simulink model "teng_sw_idc"  (R2016a)
settings: Solver=VariableStepAuto  StartTime=0.0  StopTime=5  RelTol=1e-3
libraries: fl_lib x7, elec_lib x5, nesl_utility x5, simulink x2
settings Model: Creator=mugino  LastModifiedBy=mugino
settings SolverCC: AlgebraicLoopSolver=LineSearch

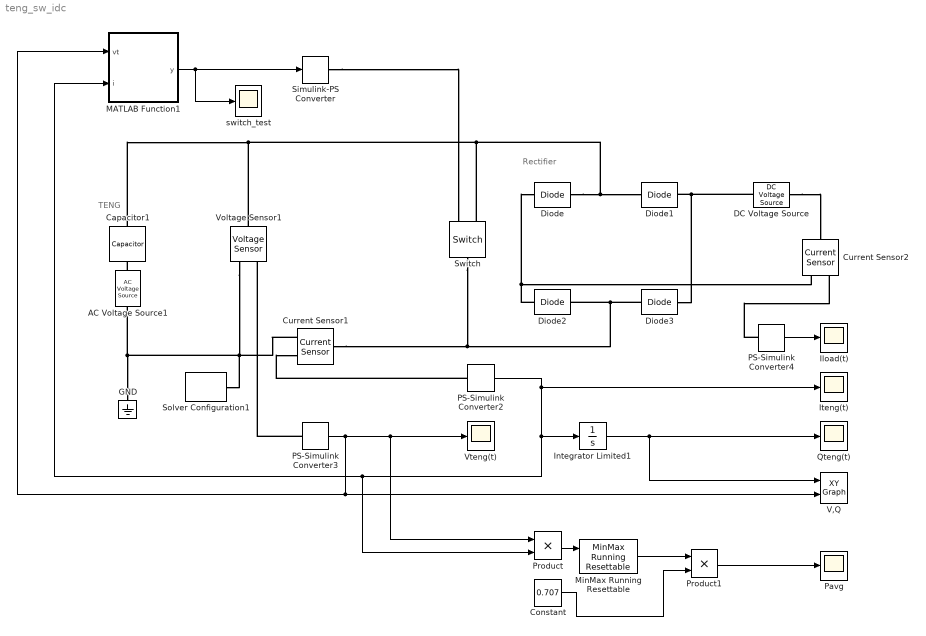
== system teng_sw_idc ==
  note: Rectifier
  note: TENG
  AC Voltage Source1 : fl_lib/Electrical/Electrical Sources/AC Voltage Source  amp=140 V  shift=90 deg  frequency=1 Hz  omega=0 rad/s
  Capacitor1 : elec_lib/Passive Devices/Capacitor  enable_table=0  c=2e-10 F  Cvec=[ 1e-5 1e-6 ] F  Vvec=[ 0 10 ] V  CV_table_symmetry=1  C_tol=5  enable_C_tol=0  tol_distribution=1  nSigma=4  r=60 MOhm  g=0 1/Ohm  initV=0 V  enable_operating_limits=0  operating_limit_action=2  max_working_voltage_range=[ -25 25 ] V  power_rating=1 W  enable_faults=0  fault_action=1  Cscale_faulted=100  R_faulted=0.001 Ohm  G_faulted=0 1/Ohm  tau_fault=0.001 s  enable_temporal_fault=0  t_fault=1 s  enable_behavioral_fault=0  max_permissible_voltage_range=[ -100 100 ] V  t_fail_on_voltage=1 s
  Constant : Constant  Value=0.707
  Current Sensor1 : fl_lib/Electrical/Electrical Sensors/Current Sensor
  Current Sensor2 : fl_lib/Electrical/Electrical Sensors/Current Sensor
  DC Voltage Source : fl_lib/Electrical/Electrical Sources/DC Voltage Source  v0=60 V
  Diode{,1..3} (4 alike) : elec_lib/Semiconductor Devices/Diode  ModelType=3  Vf=0.7 V  Ron=0.3 Ohm  Goff=1e-8 S  Rz=0.3 Ohm  Vz=50 V  C_PWL=5 pF  prmExp=1  I12=[ 0.0137 0.545 ] A  V12=[ 0.6 0.7 ] V  I1=0.0137 A  V1=0.6 V  RS=0.01 Ohm  IS=1e-12 A  Tmeas=25 degC  ec=1  BV=Inf V  C_param=1  CJ0=5 pF  VJ=1 V  Mgrad=0.5  Vvec=[ 0.1 10 100 ] V  Cvec=[ 3.5 1 0.4 ] pF  FC=0.5  Q_param=1  Irrm=-7.15 A  iF=4 A  didt=-750 A/us  trr=115 ns  TT=50 ns  tau=100 ns  T_param=1  IS_T2=1.25e-7 A  I1_T2=0.245 A  V1_T2=0.5 V  Tmeas2=125 degC  EG_param=1  EG=1.11 eV  XTI_param=1  XTI=3  dBVdT=0 V/K  Tdevice=25 degC  Rth=[ 0 10 ] K/W  thermal_mass_parameterization=1  thermal_mass=[ 0 1 ] J/K  thermal_time_constant=[ 0 10 ] s  thermal_mass_initial_temperatures=[ 25 25 ] degC
  GND : fl_lib/Electrical/Electrical Elements/Electrical Reference
  Iload(t) : Scope
  Integrator Limited1 : Integrator  LimitOutput=on  UpperSaturationLimit=1  LowerSaturationLimit=0
  Iteng(t) : Scope
  MATLAB Function1 : MATLAB Function  TreatAsAtomicUnit=on
  MinMax Running Resettable : simulink/Math Operations/MinMax Running Resettable  Function=max  vinit=0.0
  PS-Simulink Converter2 : nesl_utility/PS-Simulink Converter  PhysicalDomain=network_engine_domain  SubClassName=ps_output  LeftPortType=input  RightPortType=output  PseudoPeriodic=off  Frequencies=[]  Unit=A  AffineConversion=off
  PS-Simulink Converter3 : nesl_utility/PS-Simulink Converter  PhysicalDomain=network_engine_domain  SubClassName=ps_output  LeftPortType=input  RightPortType=output  PseudoPeriodic=off  Frequencies=[]  Unit=V  AffineConversion=off
  PS-Simulink Converter4 : nesl_utility/PS-Simulink Converter  PhysicalDomain=network_engine_domain  SubClassName=ps_output  LeftPortType=input  RightPortType=output  PseudoPeriodic=off  Frequencies=[]  Unit=A  AffineConversion=off
  "Pavg " : Scope
  Product : Product
  Product1 : Product
  Qteng(t) : Scope
  Simulink-PS Converter : nesl_utility/Simulink-PS Converter  PhysicalDomain=network_engine_domain  SubClassName=ps_input  LeftPortType=input  RightPortType=output  PseudoPeriodic=off  Frequencies=[]  NoiseDistribution=none  NoiseParameters=[]  Unit=1  AffineConversion=off  InputFiltering=off  SimscapeFilterOrder=1  InputFilterTimeConstant=0.001  UdotUserProvided=1
  Solver Configuration1 : nesl_utility/Solver Configuration  PhysicalDomain=network_engine_domain  SubClassName=solver  LeftPortType=input  RightPortType=generic  Accelerate=off  Tones=[]  Harmonics=[]  SimulateNoise=off  Profile=off  UseLocalSampling=off  EnableSwitchedLinearOptims=on  FrequencyDomain=off  UseCCode=off  RelTol=0.001  AbsTol=1e-06  MinStep=1e-09  ToWorkspace=off  RevertToSquareIcSolve=off  NumHomotopyIterations=100  PhasorMode=off  PhasorModeNumHarmonics=1  OverrideAbsTol=off  DoDC=on  ResidualTolerance=1e-06  UseLocalSolver=on  LocalSolverChoice=NE_BACKWARD_EULER_ADVANCER  LocalSolverSampleTime=0.001  DoFixedCost=on  MaxNonlinIter=3  MaxModeIter=2  LinearAlgebra=Sparse  DelaysMemoryBudget=1024  AutomaticFiltering=on  FilteringTimeConstant=0.001
  Switch : fl_lib/Electrical/Electrical Elements/Switch  R_closed=1 Ohm  G_open=1e-9 1/Ohm  Threshold=4  i_specify=off  i_priority=None  i=0 A  v_specify=off  v_priority=None  v=0 V
  V,Q : simulink/Sinks/XY Graph  xmin=-5e-9  xmax=40e-9  ymin=-150  ymax=150  st=0
  Voltage Sensor1 : fl_lib/Electrical/Electrical Sensors/Voltage Sensor
  Vteng(t) : Scope
  "switch_test " : Scope
  wires:
  PS-Simulink Converter2/1 -> Integrator Limited1/1, MATLAB Function1/2(i), Product/2, Iteng(t)/1
  PS-Simulink Converter4/1 -> Iload(t)/1
  Integrator Limited1/1 -> V,Q/1, Qteng(t)/1
  PS-Simulink Converter3/1 -> Product/1, Vteng(t)/1, V,Q/2, MATLAB Function1/1(vt)
  MATLAB Function1/1(y) -> Simulink-PS Converter/1, "switch_test "/1
  Product/1 -> MinMax Running Resettable/1
  MinMax Running Resettable/1 -> Product1/1
  Constant/1 -> Product1/2
  Product1/1 -> "Pavg "/1
  connections:
  AC Voltage Source1/RConn1 -- GND/LConn1 -- Voltage Sensor1/RConn2 -- Current Sensor1/RConn2 -- Solver Configuration1/RConn1
  Voltage Sensor1/LConn1 -- Capacitor1/LConn1 -- Diode1/LConn1 -- Diode/RConn1 -- Switch/RConn2
  Diode2/RConn1 -- Diode3/LConn1 -- Current Sensor1/LConn1 -- Switch/LConn1
  Diode2/LConn1 -- Diode/LConn1 -- Current Sensor2/RConn2
  Diode1/RConn1 -- DC Voltage Source/LConn1 -- Diode3/RConn1
  DC Voltage Source/RConn1 -- Current Sensor2/LConn1
  PS-Simulink Converter3/LConn1 -- Voltage Sensor1/RConn1
  PS-Simulink Converter2/LConn1 -- Current Sensor1/RConn1
  Simulink-PS Converter/RConn1 -- Switch/RConn1
  PS-Simulink Converter4/LConn1 -- Current Sensor2/RConn1
  AC Voltage Source1/LConn1 -- Capacitor1/RConn1

== matlab function teng_sw_idc/MATLAB Function1 ==
  data: vt input; y output; i input
function y = teng_sw(vt,i)

if(abs(i)<6e-10)       % Idc = 0
    if(abs(vt)>0.3)    % V != 0
        y=5;
    else
        y=0;
    end 
    else
        y=0;
end

% y=5;  closed (on)
% y=0;  open   (off)
